simulink model "x4bus_model"  (R2024b)
settings: Solver=VariableStepAuto  StartTime=0.0  StopTime=4  RelTol=1e-3
InitFcn:
  |         %主电路参数
  | Vin = 800;    Vtri = 400;
  | Vg = 220;     Po = 100e3*1; Qo=0;
  | Po2 = Po;    Qo2 = 0;
  | Vg1 = Vg;
  | fline = 50;   fsw = 10e3;
  | fsample = 20e3;
  | wn = 2*pi*fline;
  | L1 = 3.2e-3;  C = 50e-6;
  | L2 = 800e-6;
  | Rcf = 0.8;
  | %% GFM1
  |         %有功功率环路参数
  | Dp = 1.59e4;  %EN 50438 要求频率变化49~51Hz
  | J = 0.081;
  |         %无功功率环路参数
  | Dq = 3210;
  | K = 7.1;
  | 
  | Rv = 0.6;Lv = 3.2e-3;
  | Kp_Vreg = 0.4;
  | Ki_Vreg = 90;
  | Kp_Ireg = 11;
  | Ki_Ireg = 0;
  | 
  | Ts = 1e-6;
  | 
  | t1 = 5;
  | t2 = 100;
  | 
  | %% GFM2
  |         %有功功率环路参数
  | Dp2 = 1.59e4;  %EN 50438 要求频率变化49~51Hz
  | J2 = 0.081;
  |         %无功功率环路参数
  | Dq2 = 3210;
  | K2 = 7.1;
  | 
  | Rv2 = 0.46;Lv2 = 0.8e-3;
  | Kp_Vreg2 = 0.3;   % 0.25
  | Ki_Vreg2 = 85;    % 80
  | Kp_Ireg2 = 11;
  | Ki_Ireg2 = 0;
undefined symbols (not defined in the file or in its folder): DiscIntNeverNeededParam, t_C, t_R
libraries: spsThreePhaseSeriesRLCBranchLib x13, spsCurrentMeasurementLib x12, spsControlledVoltageSourceLib x9, slpidlib x8, spsGroundLib x7, spsabctodq0Lib x6, spsVoltageMeasurementLib x6, spsThreePhaseBreakerLib x4, spsdq0toabcLib x3, spsFirstOrderFilterLib x2, sps_lib x1
(part 2 of 2)

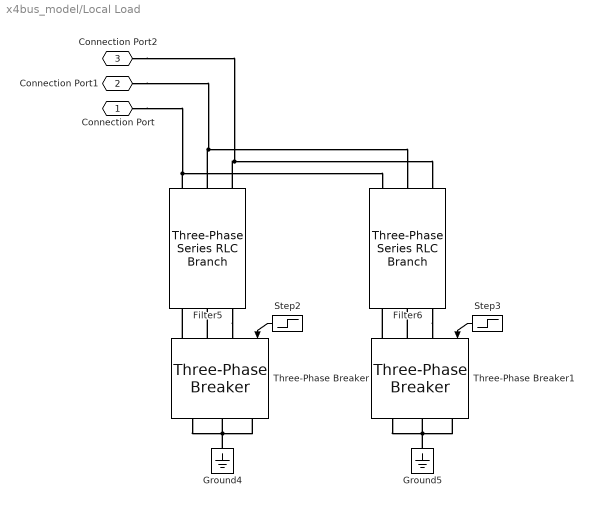
== system x4bus_model/Local Load ==
  Filter5 : spsThreePhaseSeriesRLCBranchLib/Three-Phase Series RLC Branch  LConnTagsString=A|B|C  RConnTagsString=A|B|C  BranchType=R  Resistance=100  Inductance=L2  Capacitance=50e-6  Measurements=None
  Filter6 : spsThreePhaseSeriesRLCBranchLib/Three-Phase Series RLC Branch  LConnTagsString=A|B|C  RConnTagsString=A|B|C  BranchType=C  Resistance=100  Inductance=L2  Capacitance=50e-6  Measurements=None
  Ground4 : spsGroundLib/Ground  LConnTagsString=a
  Ground5 : spsGroundLib/Ground  LConnTagsString=a
  Step2 : Step  Time=t_R  Before=1  After=0  SampleTime=0
  Step3 : Step  Time=t_C  Before=1  After=0  SampleTime=0
  Three-Phase Breaker : spsThreePhaseBreakerLib/Three-Phase Breaker  InitialState=closed  SwitchA=on  SwitchB=on  SwitchC=on  SwitchTimes="[1/60  5/60]"  External=on  BreakerResistance=0.01  SnubberResistance=1e6  SnubberCapacitance=inf  Measurements=None
  Three-Phase Breaker1 : spsThreePhaseBreakerLib/Three-Phase Breaker  InitialState=closed  SwitchA=on  SwitchB=on  SwitchC=on  SwitchTimes="[1/60  5/60]"  External=on  BreakerResistance=0.01  SnubberResistance=1e6  SnubberCapacitance=inf  Measurements=None
  Connection Port : PMIOPort  Side=Left
  Connection Port1 : PMIOPort  Port=2  Side=Left
  Connection Port2 : PMIOPort  Port=3  Side=Left
  wires:
  Step3/1 -> Three-Phase Breaker1/1
  Step2/1 -> Three-Phase Breaker/1
  connections:
  Filter5/RConn3 -- Three-Phase Breaker/LConn1
  Three-Phase Breaker/RConn2 -- Ground4/LConn1 -- Three-Phase Breaker/RConn3 -- Three-Phase Breaker/RConn1
  Ground5/LConn1 -- Three-Phase Breaker1/RConn3 -- Three-Phase Breaker1/RConn2 -- Three-Phase Breaker1/RConn1
  Three-Phase Breaker/LConn2 -- Filter5/RConn2
  Three-Phase Breaker/LConn3 -- Filter5/RConn1
  Filter5/LConn2 -- Connection Port1/RConn1 -- Filter6/LConn2
  Filter5/LConn3 -- Connection Port2/RConn1 -- Filter6/LConn3
  Filter5/LConn1 -- Connection Port/RConn1 -- Filter6/LConn1
  Three-Phase Breaker1/LConn2 -- Filter6/RConn2
  Three-Phase Breaker1/LConn3 -- Filter6/RConn1
  Filter6/RConn3 -- Three-Phase Breaker1/LConn1

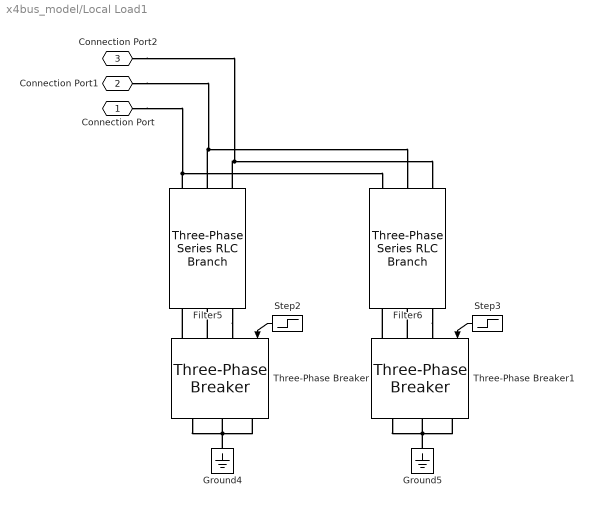
== system x4bus_model/Local Load1 ==
  Filter5 : spsThreePhaseSeriesRLCBranchLib/Three-Phase Series RLC Branch  LConnTagsString=A|B|C  RConnTagsString=A|B|C  BranchType=R  Resistance=100  Inductance=L2  Capacitance=50e-6  Measurements=None
  Filter6 : spsThreePhaseSeriesRLCBranchLib/Three-Phase Series RLC Branch  LConnTagsString=A|B|C  RConnTagsString=A|B|C  BranchType=C  Resistance=100  Inductance=L2  Capacitance=50e-6  Measurements=None
  Ground4 : spsGroundLib/Ground  LConnTagsString=a
  Ground5 : spsGroundLib/Ground  LConnTagsString=a
  Step2 : Step  Time=999  Before=1  After=0  SampleTime=0
  Step3 : Step  Time=999  Before=1  After=0  SampleTime=0
  Three-Phase Breaker : spsThreePhaseBreakerLib/Three-Phase Breaker  InitialState=closed  SwitchA=on  SwitchB=on  SwitchC=on  SwitchTimes="[1/60  5/60]"  External=on  BreakerResistance=0.01  SnubberResistance=1e6  SnubberCapacitance=inf  Measurements=None
  Three-Phase Breaker1 : spsThreePhaseBreakerLib/Three-Phase Breaker  InitialState=closed  SwitchA=on  SwitchB=on  SwitchC=on  SwitchTimes="[1/60  5/60]"  External=on  BreakerResistance=0.01  SnubberResistance=1e6  SnubberCapacitance=inf  Measurements=None
  Connection Port : PMIOPort  Side=Left
  Connection Port1 : PMIOPort  Port=2  Side=Left
  Connection Port2 : PMIOPort  Port=3  Side=Left
  wires:
  Step2/1 -> Three-Phase Breaker/1
  Step3/1 -> Three-Phase Breaker1/1
  connections:
  Filter6/RConn3 -- Three-Phase Breaker1/LConn1
  Three-Phase Breaker1/LConn3 -- Filter6/RConn1
  Three-Phase Breaker1/LConn2 -- Filter6/RConn2
  Connection Port/RConn1 -- Filter5/LConn1 -- Filter6/LConn1
  Connection Port2/RConn1 -- Filter5/LConn3 -- Filter6/LConn3
  Connection Port1/RConn1 -- Filter5/LConn2 -- Filter6/LConn2
  Three-Phase Breaker/LConn3 -- Filter5/RConn1
  Three-Phase Breaker/LConn2 -- Filter5/RConn2
  Three-Phase Breaker1/RConn2 -- Three-Phase Breaker1/RConn1 -- Ground5/LConn1 -- Three-Phase Breaker1/RConn3
  Ground4/LConn1 -- Three-Phase Breaker/RConn2 -- Three-Phase Breaker/RConn1 -- Three-Phase Breaker/RConn3
  Filter5/RConn3 -- Three-Phase Breaker/LConn1

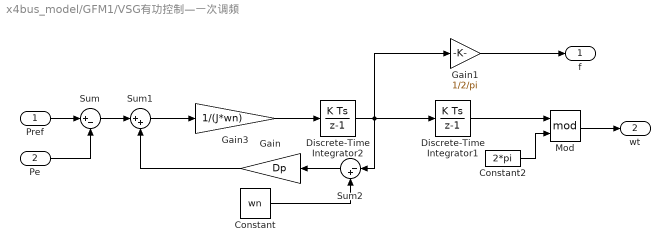
== system x4bus_model/GFM1/VSG有功控制—一次调频 ==
  Pref : Inport
  Pe : Inport  Port=2
  Constant : Constant  Value=wn
  Constant2 : Constant  Value=2*pi
  Discrete-Time Integrator1 : DiscreteIntegrator  SampleTime=-1  ICPrevOutput=DiscIntNeverNeededParam  ICPrevScaledInput=DiscIntNeverNeededParam
  Discrete-Time Integrator2 : DiscreteIntegrator  SampleTime=-1  ICPrevOutput=DiscIntNeverNeededParam  ICPrevScaledInput=DiscIntNeverNeededParam
  Gain : Gain  Gain=Dp
  Gain1 : Gain  Gain=1/2/pi
  Gain3 : Gain  Gain=1/(J*wn)
  Mod : Math  Operator=mod
  Sum : Sum  Inputs=|+-
  Sum1 : Sum  Inputs=|++
  Sum2 : Sum  Inputs=|-+
  f : Outport
  wt : Outport  Port=2
  wires:
  Sum/1 -> Sum1/1
  Sum1/1 -> Gain3/1
  Gain3/1 -> Discrete-Time Integrator2/1
  Gain1/1 -> f/1
  Discrete-Time Integrator1/1 -> Mod/1
  Constant/1 -> Sum2/2
  Constant2/1 -> Mod/2
  Pe/1 -> Sum/2
  Gain/1 -> Sum1/2
  Pref/1 -> Sum/1
  Discrete-Time Integrator2/1 -> Gain1/1, Sum2/1, Discrete-Time Integrator1/1
  Mod/1 -> wt/1
  Sum2/1 -> Gain/1

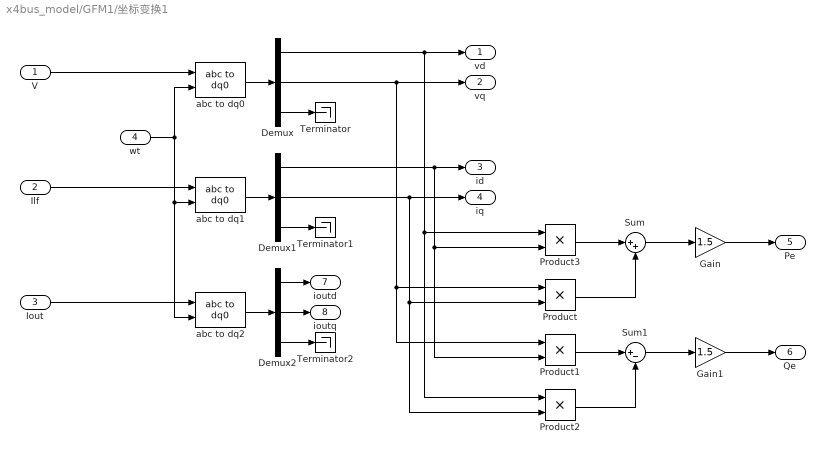
== system x4bus_model/GFM1/坐标变换1 ==
  V : Inport
  Ilf : Inport  Port=2
  Iout : Inport  Port=3
  wt : Inport  Port=4
  Demux : Demux  Outputs=3
  Demux1 : Demux  Outputs=3
  Demux2 : Demux  Outputs=3
  Gain : Gain  Gain=1.5
  Gain1 : Gain  Gain=1.5
  Product{,1..3} (4 alike) : Product
  Sum : Sum  Inputs=|++
  Sum1 : Sum  Inputs=|+-
  Terminator : Terminator
  Terminator1 : Terminator
  Terminator2 : Terminator
  abc to dq0 : spsabctodq0Lib/abc to dq0  Alignment=90 degrees behind phase A axis
  abc to dq1 : spsabctodq0Lib/abc to dq0  Alignment=90 degrees behind phase A axis
  abc to dq2 : spsabctodq0Lib/abc to dq0  Alignment=90 degrees behind phase A axis
  vd : Outport
  vq : Outport  Port=2
  id : Outport  Port=3
  iq : Outport  Port=4
  Pe : Outport  Port=5
  Qe : Outport  Port=6
  ioutd : Outport  Port=7
  ioutq : Outport  Port=8
  wires:
  Demux/1 -> Product2/1, Product3/1, vd/1
  abc to dq0/1 -> Demux/1
  Ilf/1 -> abc to dq1/1
  abc to dq1/1 -> Demux1/1
  Demux1/3 -> Terminator1/1
  Demux1/1 -> Product1/2, Product3/2, id/1
  Demux1/2 -> Product2/2, Product/2, iq/1
  Demux/2 -> Product1/1, Product/1, vq/1
  Demux/3 -> Terminator/1
  V/1 -> abc to dq0/1
  Product3/1 -> Sum/1
  Product/1 -> Sum/2
  Sum/1 -> Gain/1
  Gain/1 -> Pe/1
  Sum1/1 -> Gain1/1
  Product2/1 -> Sum1/2
  Product1/1 -> Sum1/1
  Gain1/1 -> Qe/1
  wt/1 -> abc to dq0/2, abc to dq2/2, abc to dq1/2
  abc to dq2/1 -> Demux2/1
  Iout/1 -> abc to dq2/1
  Demux2/3 -> Terminator2/1
  Demux2/1 -> ioutd/1
  Demux2/2 -> ioutq/1

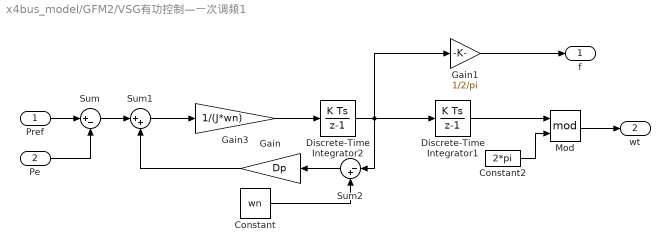
== system x4bus_model/GFM2/VSG有功控制—一次调频1 ==
  Pref : Inport
  Pe : Inport  Port=2
  Constant : Constant  Value=wn
  Constant2 : Constant  Value=2*pi
  Discrete-Time Integrator1 : DiscreteIntegrator  SampleTime=-1  ICPrevOutput=DiscIntNeverNeededParam  ICPrevScaledInput=DiscIntNeverNeededParam
  Discrete-Time Integrator2 : DiscreteIntegrator  SampleTime=-1  ICPrevOutput=DiscIntNeverNeededParam  ICPrevScaledInput=DiscIntNeverNeededParam
  Gain : Gain  Gain=Dp
  Gain1 : Gain  Gain=1/2/pi
  Gain3 : Gain  Gain=1/(J*wn)
  Mod : Math  Operator=mod
  Sum : Sum  Inputs=|+-
  Sum1 : Sum  Inputs=|++
  Sum2 : Sum  Inputs=|-+
  f : Outport
  wt : Outport  Port=2
  wires:
  Sum2/1 -> Gain/1
  Mod/1 -> wt/1
  Discrete-Time Integrator2/1 -> Discrete-Time Integrator1/1, Sum2/1, Gain1/1
  Pref/1 -> Sum/1
  Gain/1 -> Sum1/2
  Pe/1 -> Sum/2
  Constant2/1 -> Mod/2
  Constant/1 -> Sum2/2
  Discrete-Time Integrator1/1 -> Mod/1
  Gain1/1 -> f/1
  Gain3/1 -> Discrete-Time Integrator2/1
  Sum1/1 -> Gain3/1
  Sum/1 -> Sum1/1

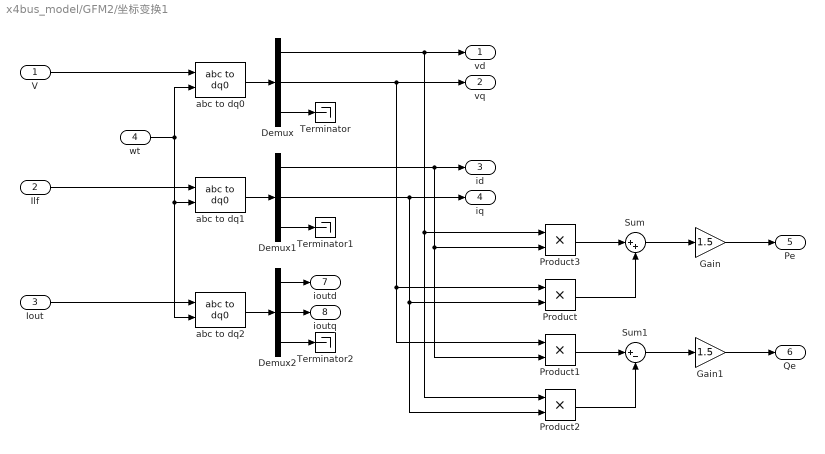
== system x4bus_model/GFM2/坐标变换1 ==
  V : Inport
  Ilf : Inport  Port=2
  Iout : Inport  Port=3
  wt : Inport  Port=4
  Demux : Demux  Outputs=3
  Demux1 : Demux  Outputs=3
  Demux2 : Demux  Outputs=3
  Gain : Gain  Gain=1.5
  Gain1 : Gain  Gain=1.5
  Product{,1..3} (4 alike) : Product
  Sum : Sum  Inputs=|++
  Sum1 : Sum  Inputs=|+-
  Terminator : Terminator
  Terminator1 : Terminator
  Terminator2 : Terminator
  abc to dq0 : spsabctodq0Lib/abc to dq0  Alignment=90 degrees behind phase A axis
  abc to dq1 : spsabctodq0Lib/abc to dq0  Alignment=90 degrees behind phase A axis
  abc to dq2 : spsabctodq0Lib/abc to dq0  Alignment=90 degrees behind phase A axis
  vd : Outport
  vq : Outport  Port=2
  id : Outport  Port=3
  iq : Outport  Port=4
  Pe : Outport  Port=5
  Qe : Outport  Port=6
  ioutd : Outport  Port=7
  ioutq : Outport  Port=8
  wires:
  Demux2/2 -> ioutq/1
  Demux2/1 -> ioutd/1
  Demux2/3 -> Terminator2/1
  Iout/1 -> abc to dq2/1
  abc to dq2/1 -> Demux2/1
  wt/1 -> abc to dq1/2, abc to dq2/2, abc to dq0/2
  Gain1/1 -> Qe/1
  Product1/1 -> Sum1/1
  Product2/1 -> Sum1/2
  Sum1/1 -> Gain1/1
  Gain/1 -> Pe/1
  Sum/1 -> Gain/1
  Product/1 -> Sum/2
  Product3/1 -> Sum/1
  V/1 -> abc to dq0/1
  Demux/3 -> Terminator/1
  Demux/2 -> vq/1, Product/1, Product1/1
  Demux1/2 -> iq/1, Product/2, Product2/2
  Demux1/1 -> id/1, Product3/2, Product1/2
  Demux1/3 -> Terminator1/1
  abc to dq1/1 -> Demux1/1
  Ilf/1 -> abc to dq1/1
  abc to dq0/1 -> Demux/1
  Demux/1 -> vd/1, Product3/1, Product2/1
